simulink library "RW_assembly_simple_lib"  (R2016b)
settings: Solver=VariableStepAuto  StartTime=0.0  StopTime=10.0  RelTol=1e-3
undefined symbols (not defined in the file or in its folder): fsw_params
libraries: simulink x3, aerolibactuator x3
settings Model: Creator=taylorreynolds  LastModifiedBy=evich

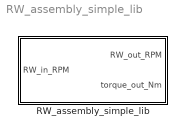
== system RW_assembly_simple_lib ==
  RW_assembly_simple_lib : Subsystem  mask{natural_frequency=100, damping_ratio=1, max_rate=100}
      mask prompts: natural_frequency "aeroblks:aeroblkactuator:blockNonlinearSecondOrderActuatorParamNaturalfrequency"; damping_ratio "aeroblks:aeroblkactuator:blockNonlinearSecondOrderActuatorParamDampingratio"; max_rate "aeroblks:aeroblkactuator:blockNonlinearSecondOrderActuatorParamRatelimit"
      mask TypeOptions natural_frequency: Nonlinear Second-Order Actuator/wn_fin | Nonlinear Second-Order Actuator1/wn_fin | Nonlinear Second-Order Actuator2/wn_fin
      mask TypeOptions damping_ratio: Nonlinear Second-Order Actuator/z_fin | Nonlinear Second-Order Actuator1/z_fin | Nonlinear Second-Order Actuator2/z_fin
      mask TypeOptions max_rate: Nonlinear Second-Order Actuator/fin_maxrate | Nonlinear Second-Order Actuator1/fin_maxrate | Nonlinear Second-Order Actuator2/fin_maxrate

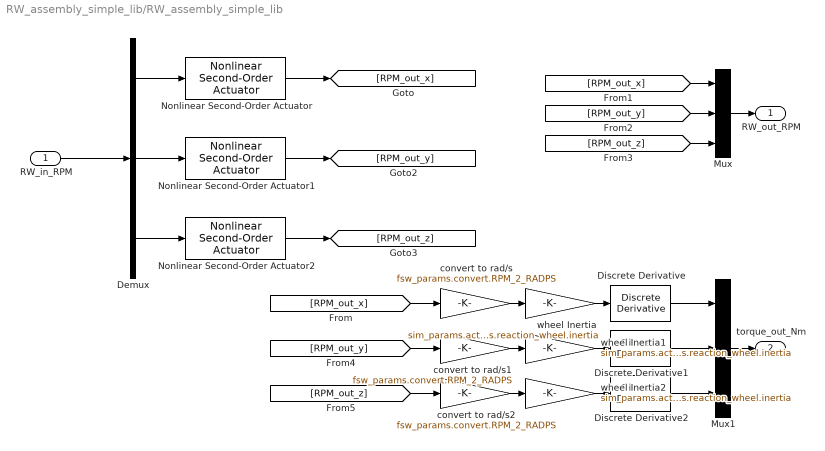
== system RW_assembly_simple_lib/RW_assembly_simple_lib ==
  RW_in_RPM : Inport
  Demux : Demux  Outputs=3
  Discrete Derivative : simulink/Discrete/Discrete Derivative  gainval=1.0  ICPrevScaledInput=sim_params.actuators.reaction_wheel.ic.deriv1  OutMin=[]  OutMax=[]  OutDataType=fixdt(1, 16)  OutScaling=2^-10  DoSatur=off
  Discrete Derivative1 : simulink/Discrete/Discrete Derivative  gainval=1.0  ICPrevScaledInput=sim_params.actuators.reaction_wheel.ic.deriv1  OutMin=[]  OutMax=[]  OutDataType=fixdt(1, 16)  OutScaling=2^-10  DoSatur=off
  Discrete Derivative2 : simulink/Discrete/Discrete Derivative  gainval=1.0  ICPrevScaledInput=sim_params.actuators.reaction_wheel.ic.deriv1  OutMin=[]  OutMax=[]  OutDataType=fixdt(1, 16)  OutScaling=2^-10  DoSatur=off
  Mux : Mux  Inputs=3
  Mux1 : Mux  Inputs=3
  Nonlinear Second-Order Actuator : aerolibactuator/Nonlinear Second-Order Actuator  wn_fin=natural_frequency  z_fin=damping_ratio  fin_max=inf  fin_min=-inf  fin_maxrate=max_rate  fin_act_0=0  fin_act_vel=0
  Nonlinear Second-Order Actuator1 : aerolibactuator/Nonlinear Second-Order Actuator  wn_fin=natural_frequency  z_fin=damping_ratio  fin_max=inf  fin_min=-inf  fin_maxrate=max_rate  fin_act_0=0  fin_act_vel=0
  Nonlinear Second-Order Actuator2 : aerolibactuator/Nonlinear Second-Order Actuator  wn_fin=natural_frequency  z_fin=damping_ratio  fin_max=inf  fin_min=-inf  fin_maxrate=max_rate  fin_act_0=0  fin_act_vel=0
  convert to rad/s : Gain  Gain=fsw_params.convert.RPM_2_RADPS
  convert to rad/s1 : Gain  Gain=fsw_params.convert.RPM_2_RADPS
  convert to rad/s2 : Gain  Gain=fsw_params.convert.RPM_2_RADPS
  wheel Inertia : Gain  Gain=sim_params.actuators.reaction_wheel.inertia
  wheel Inertia1 : Gain  Gain=sim_params.actuators.reaction_wheel.inertia
  wheel Inertia2 : Gain  Gain=sim_params.actuators.reaction_wheel.inertia
  RW_out_RPM : Outport
  torque_out_Nm : Outport  Port=2
  wires:
  RW_in_RPM/1 -> Demux/1
  Demux/1 -> Nonlinear Second-Order Actuator/1
  Demux/2 -> Nonlinear Second-Order Actuator1/1
  Demux/3 -> Nonlinear Second-Order Actuator2/1
  Nonlinear Second-Order Actuator/1 -> [RPM_out_x]
  Discrete Derivative/1 -> Mux1/1
  wheel Inertia/1 -> Discrete Derivative/1
  convert to rad/s/1 -> wheel Inertia/1
  Nonlinear Second-Order Actuator1/1 -> [RPM_out_y]
  Nonlinear Second-Order Actuator2/1 -> [RPM_out_z]
  [RPM_out_x] -> convert to rad/s/1
  [RPM_out_x] -> Mux/1
  [RPM_out_y] -> Mux/2
  [RPM_out_z] -> Mux/3
  Mux/1 -> RW_out_RPM/1
  Discrete Derivative1/1 -> Mux1/2
  wheel Inertia1/1 -> Discrete Derivative1/1
  convert to rad/s1/1 -> wheel Inertia1/1
  [RPM_out_y] -> convert to rad/s1/1
  Discrete Derivative2/1 -> Mux1/3
  wheel Inertia2/1 -> Discrete Derivative2/1
  convert to rad/s2/1 -> wheel Inertia2/1
  [RPM_out_z] -> convert to rad/s2/1
  Mux1/1 -> torque_out_Nm/1
